simulink model "tut08_01"  (R2022a)
settings: Solver=FixedStepAuto  StartTime=0.0  StopTime=30  FixedStep=0.01  MinStep=0.01  RelTol=1e-3
values from neighbouring files (symbols this model uses):
  H = 1 / 2    (= 0.5)    [tut08_01_ctrl.m]
libraries: cstblocks x2, simulink x1
settings Model: Creator=vpetrone  LastModifiedBy=Vincenzo Petrone

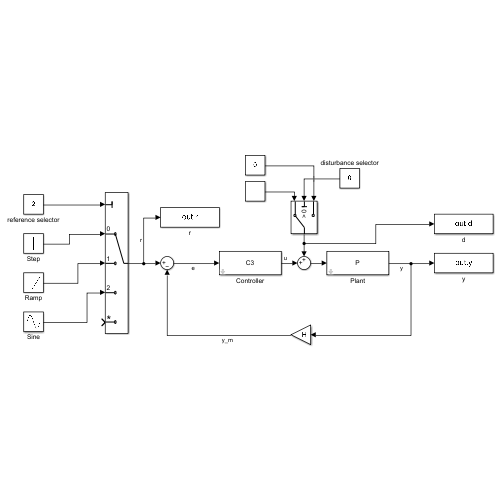
[thumbnail: Simulink's stored preview of the top-level diagram]
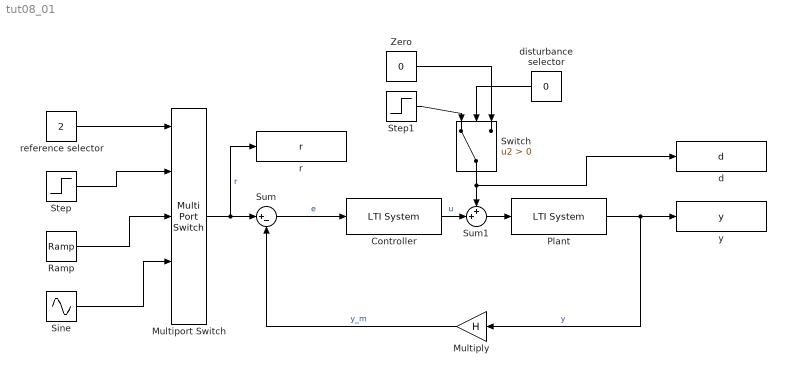
== system tut08_01 ==
  Controller : cstblocks/LTI System  sys=C3  IC=[]
  Multiply : Gain  Gain=H
  Multiport Switch : MultiPortSwitch  DataPortOrder=Zero-based contiguous  DataPortForDefault=Additional data port  zeroidx=on  SaturateOnIntegerOverflow=off  InputSameDT=off
  Plant : cstblocks/LTI System  sys=P  IC=[]
  Ramp : simulink/Sources/Ramp  slope=1  start=0  InitialOutput=0
  Sine : Sin  Amplitude=0.5  SampleTime=0
  Step : Step  Time=0  After=4  SampleTime=0
  Step1 : Step  Time=15  After=2  SampleTime=0
  Sum : Sum  Inputs=|+-
  Sum1 : Sum  Inputs=++|
  Switch : Switch  Criteria=u2 > Threshold  SaturateOnIntegerOverflow=off  InputSameDT=off
  Zero : Constant  Value=0  OutDataTypeStr=Inherit: Inherit via back propagation
  d : ToWorkspace  VariableName=d  SaveFormat=Timeseries  SampleTime=-1
  disturbance selector : Constant  Value=0
  r : ToWorkspace  VariableName=r  SaveFormat=Timeseries  SampleTime=-1
  reference selector : Constant  Value=2  SampleTime=-1
  y : ToWorkspace  VariableName=y  SaveFormat=Timeseries  SampleTime=-1
  wires:
  Controller/1 -> Sum1/2  "u"
  Plant/1 -> Multiply/1, y/1  "y"
  Sum/1 -> Controller/1  "e"
  Multiply/1 -> Sum/2  "y_m"
  Step/1 -> Multiport Switch/2
  Ramp/1 -> Multiport Switch/3
  Sine/1 -> Multiport Switch/4
  Multiport Switch/1 -> r/1, Sum/1  "r"
  reference selector/1 -> Multiport Switch/1
  Sum1/1 -> Plant/1
  Switch/1 -> d/1, Sum1/1
  Step1/1 -> Switch/1
  Zero/1 -> Switch/3
  disturbance selector/1 -> Switch/2
